simulink model "exam"  (Simulink 7.6)
settings: Solver=ode45  StartTime=0.0  StopTime=100.0  RelTol=1e-3
values from neighbouring files (symbols this model uses):
  mu = 1    [exam.m]    (also in exam1.m)
settings Model: Creator=Administrator  LastModifiedBy=Administrator

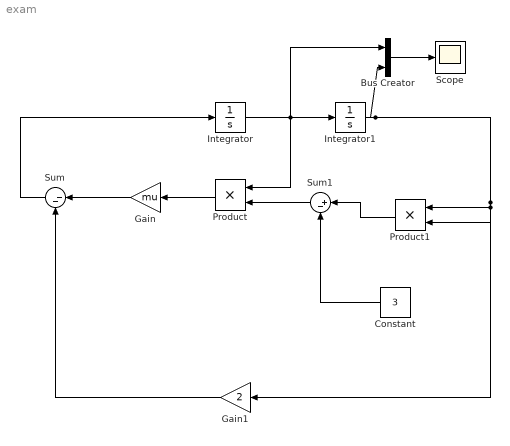
== system exam ==
  Bus Creator : BusCreator  Inputs=2
  Constant : Constant  Value=3
  Gain : Gain  Gain=mu
  Gain1 : Gain  Gain=2
  Integrator : Integrator  InitialCondition=-1
  Integrator1 : Integrator  InitialCondition=-2
  Product : Product  RndMeth=Zero
  Product1 : Product  RndMeth=Zero
  Scope : Scope
  Sum : Sum  Inputs=|--
  Sum1 : Sum  Inputs=|+-
  wires:
  Integrator/1 -> Integrator1/1, Product/1, Bus Creator/1
  Integrator1/1 -> Product1/2, Product1/1, Gain1/1, Bus Creator/2
  Constant/1 -> Sum1/2
  Product1/1 -> Sum1/1
  Sum1/1 -> Product/2
  Product/1 -> Gain/1
  Gain/1 -> Sum/1
  Gain1/1 -> Sum/2
  Sum/1 -> Integrator/1
  Bus Creator/1 -> Scope/1
